simulink model "final_quadruped_230622gimbleRF"  (R2021a)
settings: Solver=ode15s  StartTime=0.0  StopTime=10  FixedStep=1e-3  RelTol=1e-5  EnableMultiTasking=on
values from neighbouring files (symbols this model uses):
  foot_x = 8    [bipedparameters.m]    (also in fcn.m; finalrobotParameters.m; finalrobotParameters_110522.m; finalrobotParameters_140522.m)
  foot_y = 6    [bipedparameters.m]    (also in fcn.m; finalrobotParameters.m; finalrobotParameters_110522.m; finalrobotParameters_140522.m)
  foot_z = 1    [bipedparameters.m]    (also in fcn.m; finalrobotParameters.m; finalrobotParameters_110522.m; finalrobotParameters_140522.m)
  height_plane = 0.025    [bipedparameters.m]    (also in finalrobotParameters.m; finalrobotParameters_110522.m; finalrobotParameters_140522.m; finalrobotParameters_240522.m)
  kd_ankle = 1000    [bipedparameters.m]    (also in finalrobotParameters_240522.m)
  kd_hip = 1000    [bipedparameters.m]    (also in finalrobotParameters_240522.m)
  kd_knee = 1000    [bipedparameters.m]    (also in finalrobotParameters_240522.m)
  ki_ankle = 1000    [bipedparameters.m]    (also in finalrobotParameters_240522.m)
  ki_hip = 1000    [bipedparameters.m]    (also in finalrobotParameters_240522.m)
  ki_knee = 2000    [bipedparameters.m]    (also in finalrobotParameters_240522.m)
  kp_ankle = 1000    [bipedparameters.m]    (also in finalrobotParameters_240522.m)
  kp_hip = 1000    [bipedparameters.m]    (also in finalrobotParameters_240522.m)
  kp_knee = 2000    [bipedparameters.m]    (also in finalrobotParameters_240522.m)
  lower_leg_length = 10    [bipedparameters.m]    (also in fcn.m; finalrobotParameters.m; finalrobotParameters_110522.m; finalrobotParameters_140522.m)
  m_ll = density*leg_radius*leg_radius*lower_leg_length*3.141592653589*0.01*0.01*0.01    (= 0.0176714586764)    [bipedparameters.m]    (also in fcn.m; finalrobotParameters_140522.m; finalrobotParameters_240522.m; hdotlb.m)
  m_ul = density*leg_radius*leg_radius*upper_leg_length*3.141592653589*0.01*0.01*0.01    (= 0.0176714586764)    [bipedparameters.m]    (also in fcn.m; finalrobotParameters_140522.m; finalrobotParameters_240522.m; hdotlb.m)
  plane_x = 25    [bipedparameters.m]    (also in finalrobotParameters.m; finalrobotParameters_110522.m; finalrobotParameters_140522.m; finalrobotParameters_240522.m)
  plane_y = 3    [bipedparameters.m]    (also in finalrobotParameters.m; finalrobotParameters_110522.m; finalrobotParameters_140522.m; finalrobotParameters_240522.m)
  torso_offset_x = -0.5    [bipedparameters.m]    (also in finalrobotParameters.m = 10; finalrobotParameters_110522.m = 10; finalrobotParameters_140522.m = 10; finalrobotParameters_240522.m = 10)
  torso_offset_z = -2    [bipedparameters.m]    (also in finalrobotParameters.m; finalrobotParameters_110522.m; finalrobotParameters_140522.m; finalrobotParameters_240522.m)
  torso_x = 5    [bipedparameters.m]    (also in fcn.m = 25; finalrobotParameters.m = 25; finalrobotParameters_110522.m = 25; finalrobotParameters_140522.m = 25)
  torso_y = 10    [bipedparameters.m]    (also in fcn.m = 16; finalrobotParameters.m = 16; finalrobotParameters_110522.m = 16; finalrobotParameters_140522.m = 16)
  torso_z = 8    [bipedparameters.m]    (also in fcn.m = 10; finalrobotParameters.m = 10; finalrobotParameters_110522.m = 10; finalrobotParameters_140522.m = 10)
  upper_leg_length = 10    [bipedparameters.m]    (also in fcn.m; finalrobotParameters.m; finalrobotParameters_110522.m; finalrobotParameters_140522.m)
undefined symbols (not defined in the file or in its folder): sigbuilder_block, X, Y, Z
libraries: nesl_utility x201, sm_lib x71, Contact_Forces_Lib x16, pid_lib x14, fl_lib x3
(part 7 of 8)

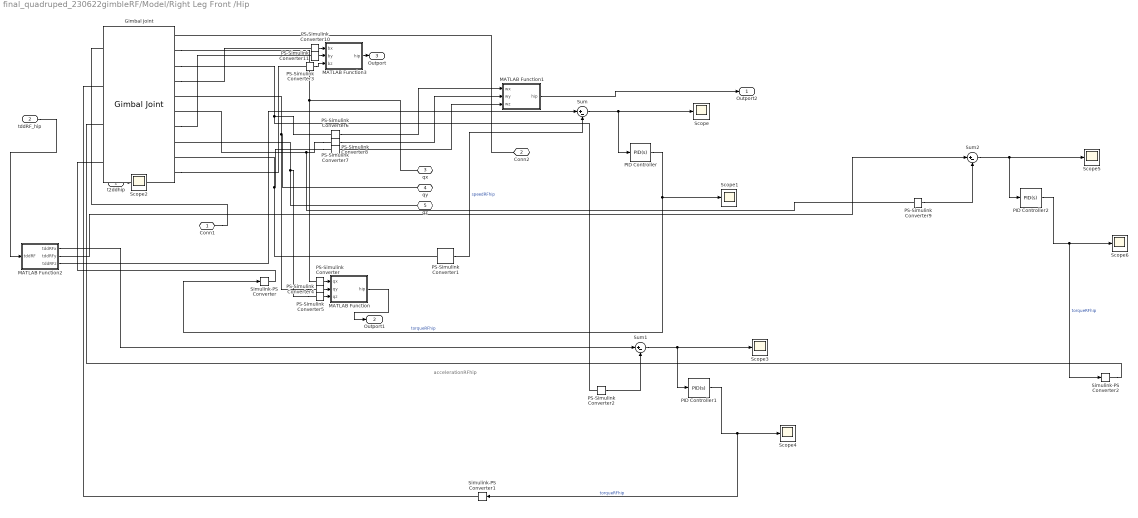
== system final_quadruped_230622gimbleRF/Model/Right Leg Front /Hip ==
  note: accelerationRFhip
  t2ddhip : Inport
  tddRF_hip : Inport  Port=2
  Gimbal Joint : sm_lib/Joints/Gimbal Joint  JointMode=Normal  SenseConstraintForce=off  SenseConstraintForceX=off  SenseConstraintForceY=off  SenseConstraintForceZ=off  SenseConstraintTorque=off  SenseConstraintTorqueX=off  SenseConstraintTorqueY=off  SenseConstraintTorqueZ=off  SenseTotalForce=off  SenseTotalForceX=off  SenseTotalForceY=off  SenseTotalForceZ=off  SenseTotalTorque=off  SenseTotalTorqueX=off  SenseTotalTorqueY=off  SenseTotalTorqueZ=off  CompositeWrenchDir=FollowerOnBase  CompositeWrenchFrame=BaseFrame  RxEquilibriumPosition=0  RxEquilibriumPositionUnits=deg  RxSpringStiffness=0  RxSpringStiffnessUnits=N*m/deg  RxDampingCoefficient=0  RxDampingCoefficientUnits=N*m/(deg/s)  RxTorqueActuationMode=InputTorque  RxMotionActuationMode=ComputedMotion  RxSensePosition=on  RxSenseVelocity=on  RxSenseAcceleration=on  RxSenseTorqueForce=off  RxSenseLowerLimitTorqueForce=off  RxSenseUpperLimitTorqueForce=off  RxLowerLimitSpecify=off  RxLowerLimitBound=-90  RxLowerLimitBoundUnits=deg  RxLowerLimitStiffness=1e4  RxLowerLimitStiffnessUnits=N*m/deg  RxLowerLimitDamping=10  RxLowerLimitDampingUnits=N*m/(deg/s)  RxLowerLimitTransitionRegionWidth=0.1  RxLowerLimitTransitionRegionWidthUnits=deg  RxUpperLimitSpecify=off  RxUpperLimitBound=90  RxUpperLimitBoundUnits=deg  RxUpperLimitStiffness=1e4  RxUpperLimitStiffnessUnits=N*m/deg  RxUpperLimitDamping=10  RxUpperLimitDampingUnits=N*m/(deg/s)  RxUpperLimitTransitionRegionWidth=0.1  RxUpperLimitTransitionRegionWidthUnits=deg  RxPositionTargetSpecify=off  RxPositionTargetPriority=High  RxPositionTargetValue=0  RxPositionTargetValueUnits=deg  RxVelocityTargetSpecify=off  RxVelocityTargetPriority=High  RxVelocityTargetValue=0  RxVelocityTargetValueUnits=deg/s  RyEquilibriumPosition=0  RyEquilibriumPositionUnits=deg  RySpringStiffness=0  RySpringStiffnessUnits=N*m/deg  RyDampingCoefficient=0  RyDampingCoefficientUnits=N*m/(deg/s)  RyTorqueActuationMode=InputTorque  RyMotionActuationMode=ComputedMotion  RySensePosition=on  RySenseVelocity=on  RySenseAcceleration=on  RySenseTorqueForce=off  RySenseLowerLimitTorqueForce=off  RySenseUpperLimitTorqueForce=off  RyLowerLimitSpecify=off  RyLowerLimitBound=-90  RyLowerLimitBoundUnits=deg  RyLowerLimitStiffness=1e4  RyLowerLimitStiffnessUnits=N*m/deg  RyLowerLimitDamping=10  RyLowerLimitDampingUnits=N*m/(deg/s)  RyLowerLimitTransitionRegionWidth=0.1  RyLowerLimitTransitionRegionWidthUnits=deg  RyUpperLimitSpecify=off  RyUpperLimitBound=90  RyUpperLimitBoundUnits=deg  RyUpperLimitStiffness=1e4  RyUpperLimitStiffnessUnits=N*m/deg  RyUpperLimitDamping=10  RyUpperLimitDampingUnits=N*m/(deg/s)  RyUpperLimitTransitionRegionWidth=0.1  RyUpperLimitTransitionRegionWidthUnits=deg  RyPositionTargetSpecify=off  RyPositionTargetPriority=High  RyPositionTargetValue=0  RyPositionTargetValueUnits=deg  RyVelocityTargetSpecify=off  RyVelocityTargetPriority=High  RyVelocityTargetValue=0  RyVelocityTargetValueUnits=deg/s  RzEquilibriumPosition=0  RzEquilibriumPositionUnits=deg  RzSpringStiffness=0  RzSpringStiffnessUnits=N*m/deg  RzDampingCoefficient=0  RzDampingCoefficientUnits=N*m/(deg/s)  RzTorqueActuationMode=InputTorque  RzMotionActuationMode=ComputedMotion  RzSensePosition=on  RzSenseVelocity=on  RzSenseAcceleration=on  RzSenseTorqueForce=off  RzSenseLowerLimitTorqueForce=off  RzSenseUpperLimitTorqueForce=off  RzLowerLimitSpecify=off  RzLowerLimitBound=-90  RzLowerLimitBoundUnits=deg  RzLowerLimitStiffness=1e4  RzLowerLimitStiffnessUnits=N*m/deg  RzLowerLimitDamping=10  RzLowerLimitDampingUnits=N*m/(deg/s)  RzLowerLimitTransitionRegionWidth=0.1  RzLowerLimitTransitionRegionWidthUnits=deg  RzUpperLimitSpecify=off  RzUpperLimitBound=90  RzUpperLimitBoundUnits=deg  RzUpperLimitStiffness=1e4  RzUpperLimitStiffnessUnits=N*m/deg  RzUpperLimitDamping=10  RzUpperLimitDampingUnits=N*m/(deg/s)  RzUpperLimitTransitionRegionWidth=0.1  RzUpperLimitTransitionRegionWidthUnits=deg  RzPositionTargetSpecify=on  RzPositionTargetPriority=Low  RzPositionTargetValue=-10  RzPositionTargetValueUnits=deg  RzVelocityTargetSpecify=on  RzVelocityTargetPriority=Low  RzVelocityTargetValue=1  RzVelocityTargetValueUnits=deg/s
  MATLAB Function : MATLAB Function  TreatAsAtomicUnit=on
  MATLAB Function1 : MATLAB Function  TreatAsAtomicUnit=on
  MATLAB Function2 : MATLAB Function  TreatAsAtomicUnit=on
  MATLAB Function3 : MATLAB Function  TreatAsAtomicUnit=on
  PID Controller : pid_lib/PID Controller  Controller=PID  Form=Parallel  TimeDomain=Continuous-time  UseExternalTs=off  SampleTime=-1  IntegratorMethod=Forward Euler  FilterMethod=Forward Euler  ControllerParametersSource=internal  P=kp_hip  I=ki_hip  D=kd_hip  UseFilter=on  N=100  TunerSelectOption=Transfer Function Based (PID Tuner App)  InitialConditionSource=internal  InitialConditionForIntegrator=0  InitialConditionForFilter=0  DifferentiatorICPrevScaledInput=0  ExternalReset=none  TrackingMode=off  Kt=1  LimitOutput=off  SatLimitsSource=internal  UpperSaturationLimit=inf  LowerSaturationLimit=-inf  LinearizeAsGain=on  AntiWindupMode=none  Kb=1  POutMin=[]  POutMax=[]  IOutMin=[]  IOutMax=[]  DOutMin=[]  DOutMax=[]  NOutMin=[]  NOutMax=[]  SumOutMin=[]  SumOutMax=[]  SaturationOutMin=[]  SaturationOutMax=[]  PParamMin=[]  PParamMax=[]  IParamMin=[]  IParamMax=[]  DParamMin=[]  DParamMax=[]  NParamMin=[]  NParamMax=[]  KbParamMin=[]  KbParamMax=[]  KtParamMin=[]  KtParamMax=[]  KbOutMin=[]  KbOutMax=[]  KtOutMin=[]  KtOutMax=[]  IntegratorOutMin=[]  IntegratorOutMax=[]  FilterOutMin=[]  FilterOutMax=[]  SumI1OutMin=[]  SumI1OutMax=[]  SumI2OutMin=[]  SumI2OutMax=[]  SumI3OutMin=[]  SumI3OutMax=[]  SumI4OutMin=[]  SumI4OutMax=[]  SumDOutMin=[]  SumDOutMax=[]  DifferentiatorOutMin=[]  DifferentiatorOutMax=[]  FilterDiffOutCoefMin=[]  FilterDiffOutCoefMax=[]  ReciprocalOutMin=[]  ReciprocalOutMax=[]  SumDenOutMin=[]  SumDenOutMax=[]  SumNumOutMin=[]  SumNumOutMax=[]  DivideOutMin=[]  DivideOutMax=[]  UdiffTsProdOutMin=[]  UdiffTsProdOutMax=[]  NTsProdOutMin=[]  NTsProdOutMax=[]  UintegralTsProdOutMin=[]  UintegralTsProdOutMax=[]  UngainTsProdOutMin=[]  UngainTsProdOutMax=[]  IntegratorContinuousStateAttributes=''  IntegratorStateMustResolveToSignalObject=off  IntegratorRTWStateStorageClass=Auto  FilterContinuousStateAttributes=''  FilterStateMustResolveToSignalObject=off  FilterRTWStateStorageClass=Auto  ParallelPVariant=InternalParameters  IdealPVariant=Disabled  IVariant=InternalParameters  DVariant=InternalParameters  IntegratorVariant=Continuous  SatVariant=Disabled  AWVariant=Passthrough  PCopyVariant=Disabled  TRVariant=Disabled  FdbkBlocksVariant=Forward  IdealPFdbkVariant=Disabled  SatFdbkVariant=Disabled  DerivativeFilterVariant=ContFilter  NVariant=InternalParameters  NCopyVariant=Disabled  FilterICVariant=InternalICsFilter  IntegratorICVariant=InternalICs  ExternalResetVariant=Disabled  TRSumVariant=Passthrough  SumFdbkVariant=Disabled  SumVariant=Sum_PID  TsampFilterVariant=InternalTs  TsampNgainVariant=Passthrough  TsampIntegralVariant=Passthrough  ExternalSaturationOutDataTypeStr=Inherit: Same as second input
  PID Controller1 : pid_lib/PID Controller  Controller=PID  Form=Parallel  TimeDomain=Continuous-time  UseExternalTs=off  SampleTime=-1  IntegratorMethod=Forward Euler  FilterMethod=Forward Euler  ControllerParametersSource=internal  P=kp_hip  I=ki_hip  D=kd_hip  UseFilter=on  N=100  TunerSelectOption=Transfer Function Based (PID Tuner App)  InitialConditionSource=internal  InitialConditionForIntegrator=0  InitialConditionForFilter=0  DifferentiatorICPrevScaledInput=0  ExternalReset=none  TrackingMode=off  Kt=1  LimitOutput=off  SatLimitsSource=internal  UpperSaturationLimit=inf  LowerSaturationLimit=-inf  LinearizeAsGain=on  AntiWindupMode=none  Kb=1  POutMin=[]  POutMax=[]  IOutMin=[]  IOutMax=[]  DOutMin=[]  DOutMax=[]  NOutMin=[]  NOutMax=[]  SumOutMin=[]  SumOutMax=[]  SaturationOutMin=[]  SaturationOutMax=[]  PParamMin=[]  PParamMax=[]  IParamMin=[]  IParamMax=[]  DParamMin=[]  DParamMax=[]  NParamMin=[]  NParamMax=[]  KbParamMin=[]  KbParamMax=[]  KtParamMin=[]  KtParamMax=[]  KbOutMin=[]  KbOutMax=[]  KtOutMin=[]  KtOutMax=[]  IntegratorOutMin=[]  IntegratorOutMax=[]  FilterOutMin=[]  FilterOutMax=[]  SumI1OutMin=[]  SumI1OutMax=[]  SumI2OutMin=[]  SumI2OutMax=[]  SumI3OutMin=[]  SumI3OutMax=[]  SumI4OutMin=[]  SumI4OutMax=[]  SumDOutMin=[]  SumDOutMax=[]  DifferentiatorOutMin=[]  DifferentiatorOutMax=[]  FilterDiffOutCoefMin=[]  FilterDiffOutCoefMax=[]  ReciprocalOutMin=[]  ReciprocalOutMax=[]  SumDenOutMin=[]  SumDenOutMax=[]  SumNumOutMin=[]  SumNumOutMax=[]  DivideOutMin=[]  DivideOutMax=[]  UdiffTsProdOutMin=[]  UdiffTsProdOutMax=[]  NTsProdOutMin=[]  NTsProdOutMax=[]  UintegralTsProdOutMin=[]  UintegralTsProdOutMax=[]  UngainTsProdOutMin=[]  UngainTsProdOutMax=[]  IntegratorContinuousStateAttributes=''  IntegratorStateMustResolveToSignalObject=off  IntegratorRTWStateStorageClass=Auto  FilterContinuousStateAttributes=''  FilterStateMustResolveToSignalObject=off  FilterRTWStateStorageClass=Auto  ParallelPVariant=InternalParameters  IdealPVariant=Disabled  IVariant=InternalParameters  DVariant=InternalParameters  IntegratorVariant=Continuous  SatVariant=Disabled  AWVariant=Passthrough  PCopyVariant=Disabled  TRVariant=Disabled  FdbkBlocksVariant=Forward  IdealPFdbkVariant=Disabled  SatFdbkVariant=Disabled  DerivativeFilterVariant=ContFilter  NVariant=InternalParameters  NCopyVariant=Disabled  FilterICVariant=InternalICsFilter  IntegratorICVariant=InternalICs  ExternalResetVariant=Disabled  TRSumVariant=Passthrough  SumFdbkVariant=Disabled  SumVariant=Sum_PID  TsampFilterVariant=InternalTs  TsampNgainVariant=Passthrough  TsampIntegralVariant=Passthrough  ExternalSaturationOutDataTypeStr=Inherit: Same as second input
  PID Controller2 : pid_lib/PID Controller  Controller=PID  Form=Parallel  TimeDomain=Continuous-time  UseExternalTs=off  SampleTime=-1  IntegratorMethod=Forward Euler  FilterMethod=Forward Euler  ControllerParametersSource=internal  P=kp_hip  I=ki_hip  D=kd_hip  UseFilter=on  N=100  TunerSelectOption=Transfer Function Based (PID Tuner App)  InitialConditionSource=internal  InitialConditionForIntegrator=0  InitialConditionForFilter=0  DifferentiatorICPrevScaledInput=0  ExternalReset=none  TrackingMode=off  Kt=1  LimitOutput=off  SatLimitsSource=internal  UpperSaturationLimit=inf  LowerSaturationLimit=-inf  LinearizeAsGain=on  AntiWindupMode=none  Kb=1  POutMin=[]  POutMax=[]  IOutMin=[]  IOutMax=[]  DOutMin=[]  DOutMax=[]  NOutMin=[]  NOutMax=[]  SumOutMin=[]  SumOutMax=[]  SaturationOutMin=[]  SaturationOutMax=[]  PParamMin=[]  PParamMax=[]  IParamMin=[]  IParamMax=[]  DParamMin=[]  DParamMax=[]  NParamMin=[]  NParamMax=[]  KbParamMin=[]  KbParamMax=[]  KtParamMin=[]  KtParamMax=[]  KbOutMin=[]  KbOutMax=[]  KtOutMin=[]  KtOutMax=[]  IntegratorOutMin=[]  IntegratorOutMax=[]  FilterOutMin=[]  FilterOutMax=[]  SumI1OutMin=[]  SumI1OutMax=[]  SumI2OutMin=[]  SumI2OutMax=[]  SumI3OutMin=[]  SumI3OutMax=[]  SumI4OutMin=[]  SumI4OutMax=[]  SumDOutMin=[]  SumDOutMax=[]  DifferentiatorOutMin=[]  DifferentiatorOutMax=[]  FilterDiffOutCoefMin=[]  FilterDiffOutCoefMax=[]  ReciprocalOutMin=[]  ReciprocalOutMax=[]  SumDenOutMin=[]  SumDenOutMax=[]  SumNumOutMin=[]  SumNumOutMax=[]  DivideOutMin=[]  DivideOutMax=[]  UdiffTsProdOutMin=[]  UdiffTsProdOutMax=[]  NTsProdOutMin=[]  NTsProdOutMax=[]  UintegralTsProdOutMin=[]  UintegralTsProdOutMax=[]  UngainTsProdOutMin=[]  UngainTsProdOutMax=[]  IntegratorContinuousStateAttributes=''  IntegratorStateMustResolveToSignalObject=off  IntegratorRTWStateStorageClass=Auto  FilterContinuousStateAttributes=''  FilterStateMustResolveToSignalObject=off  FilterRTWStateStorageClass=Auto  ParallelPVariant=InternalParameters  IdealPVariant=Disabled  IVariant=InternalParameters  DVariant=InternalParameters  IntegratorVariant=Continuous  SatVariant=Disabled  AWVariant=Passthrough  PCopyVariant=Disabled  TRVariant=Disabled  FdbkBlocksVariant=Forward  IdealPFdbkVariant=Disabled  SatFdbkVariant=Disabled  DerivativeFilterVariant=ContFilter  NVariant=InternalParameters  NCopyVariant=Disabled  FilterICVariant=InternalICsFilter  IntegratorICVariant=InternalICs  ExternalResetVariant=Disabled  TRSumVariant=Passthrough  SumFdbkVariant=Disabled  SumVariant=Sum_PID  TsampFilterVariant=InternalTs  TsampNgainVariant=Passthrough  TsampIntegralVariant=Passthrough  ExternalSaturationOutDataTypeStr=Inherit: Same as second input
  PS-Simulink Converter{,2..11} (11 alike) : nesl_utility/PS-Simulink Converter  PhysicalDomain=network_engine_domain  SubClassName=ps_output  LeftPortType=input  RightPortType=output  PseudoPeriodic=off  Frequencies=[]  Unit=inherit  AffineConversion=off
      settings: SourceProductBaseCode=PW,SS
  PS-Simulink Converter1 : nesl_utility/PS-Simulink Converter  PhysicalDomain=network_engine_domain  SubClassName=ps_output  LeftPortType=input  RightPortType=output  PseudoPeriodic=off  Frequencies=[]  Unit=1  AffineConversion=off
      settings: SourceProductBaseCode=PW,SS
  Scope{,1..6} (7 alike) : Scope
  Simulink-PS Converter : nesl_utility/Simulink-PS Converter  PhysicalDomain=network_engine_domain  SubClassName=ps_input  LeftPortType=input  RightPortType=output  PseudoPeriodic=off  Frequencies=[]  NoiseDistribution=none  NoiseParameters=[]  Unit=1  AffineConversion=off  FilteringAndDerivatives=provide  SimscapeFilterOrder=1  InputFilterTimeConstant=0.001  UdotUserProvided=0
      settings: SourceProductBaseCode=PW,SS
  Simulink-PS Converter1 : nesl_utility/Simulink-PS Converter  PhysicalDomain=network_engine_domain  SubClassName=ps_input  LeftPortType=input  RightPortType=output  PseudoPeriodic=off  Frequencies=[]  NoiseDistribution=none  NoiseParameters=[]  Unit=1  AffineConversion=off  FilteringAndDerivatives=provide  SimscapeFilterOrder=1  InputFilterTimeConstant=0.001  UdotUserProvided=0
      settings: SourceProductBaseCode=PW,SS
  Simulink-PS Converter2 : nesl_utility/Simulink-PS Converter  PhysicalDomain=network_engine_domain  SubClassName=ps_input  LeftPortType=input  RightPortType=output  PseudoPeriodic=off  Frequencies=[]  NoiseDistribution=none  NoiseParameters=[]  Unit=1  AffineConversion=off  FilteringAndDerivatives=provide  SimscapeFilterOrder=1  InputFilterTimeConstant=0.001  UdotUserProvided=0
      settings: SourceProductBaseCode=PW,SS
  Sum : Sum  Inputs=|+-
  Sum1 : Sum  Inputs=|+-
  Sum2 : Sum  Inputs=|+-
  Conn1 : PMIOPort  Side=Left
  Conn2 : PMIOPort  Port=2  Side=Right
  qx : PMIOPort  Port=3  Side=Right
  qy : PMIOPort  Port=4  Side=Right
  qz : PMIOPort  Port=5  Side=Right
  Outport2 : Outport
  Outport1 : Outport  Port=2
  Outport : Outport  Port=3
  wires:
  PS-Simulink Converter1/1 -> Sum/2  "speedRFhip"
  Sum/1 -> PID Controller/1, Scope/1
  PID Controller/1 -> Scope1/1, Simulink-PS Converter/1  "torqueRFhip"
  MATLAB Function1/1(hip) -> Outport2/1
  t2ddhip/1 -> Scope2/1
  PS-Simulink Converter/1 -> MATLAB Function/1(qx)
  PS-Simulink Converter4/1 -> MATLAB Function/2(qy)
  PS-Simulink Converter5/1 -> MATLAB Function/3(qz)
  MATLAB Function/1(hip) -> Outport1/1
  PS-Simulink Converter6/1 -> MATLAB Function1/1(wx)
  PS-Simulink Converter7/1 -> MATLAB Function1/2(wy)
  PS-Simulink Converter8/1 -> MATLAB Function1/3(wz)
  tddRF_hip/1 -> MATLAB Function2/1(tddRF)
  PID Controller1/1 -> Simulink-PS Converter1/1, Scope4/1  "torqueRFhip"
  Sum1/1 -> PID Controller1/1, Scope3/1
  MATLAB Function2/1(tddRFx) -> Sum1/1
  PS-Simulink Converter2/1 -> Sum1/2
  MATLAB Function2/3(tddRFz) -> Sum/1
  PID Controller2/1 -> Simulink-PS Converter2/1, Scope6/1  "torqueRFhip"
  Sum2/1 -> PID Controller2/1, Scope5/1
  MATLAB Function2/2(tddRFy) -> Sum2/1
  PS-Simulink Converter9/1 -> Sum2/2
  PS-Simulink Converter10/1 -> MATLAB Function3/1(bx)
  PS-Simulink Converter3/1 -> MATLAB Function3/3(bz)
  PS-Simulink Converter11/1 -> MATLAB Function3/2(by)
  MATLAB Function3/1(hip) -> Outport/1
  connections:
  Conn2/RConn1 -- Gimbal Joint/RConn1
  Conn1/RConn1 -- Gimbal Joint/LConn1
  Gimbal Joint/RConn2 -- qx/RConn1 -- PS-Simulink Converter/LConn1
  PS-Simulink Converter4/LConn1 -- Gimbal Joint/RConn5 -- qy/RConn1
  PS-Simulink Converter5/LConn1 -- Gimbal Joint/RConn8 -- qz/RConn1
  Gimbal Joint/RConn3 -- PS-Simulink Converter2/LConn1 -- PS-Simulink Converter6/LConn1
  PS-Simulink Converter7/LConn1 -- Gimbal Joint/RConn6 -- PS-Simulink Converter9/LConn1
  PS-Simulink Converter8/LConn1 -- Gimbal Joint/RConn9 -- PS-Simulink Converter1/LConn1
  Simulink-PS Converter1/RConn1 -- Gimbal Joint/LConn2
  Simulink-PS Converter2/RConn1 -- Gimbal Joint/LConn3
  Simulink-PS Converter/RConn1 -- Gimbal Joint/LConn4
  Gimbal Joint/RConn4 -- PS-Simulink Converter10/LConn1
  Gimbal Joint/RConn7 -- PS-Simulink Converter11/LConn1
  Gimbal Joint/RConn10 -- PS-Simulink Converter3/LConn1

== system final_quadruped_230622gimbleRF/Model/Right Leg Front /Knee ==
  note: accelerationRFknee
  note: Meas for knee
  tddRF_knee : Inport
  t2ddknee : Inport  Port=2
  Bus Creator : BusCreator  Inputs=3
  Knee joint : sm_lib/Joints/Revolute Joint  JointMode=Normal  SenseConstraintForce=off  SenseConstraintForceX=off  SenseConstraintForceY=off  SenseConstraintForceZ=off  SenseConstraintTorque=off  SenseConstraintTorqueX=off  SenseConstraintTorqueY=off  SenseConstraintTorqueZ=off  SenseTotalForce=off  SenseTotalForceX=off  SenseTotalForceY=off  SenseTotalForceZ=off  SenseTotalTorque=off  SenseTotalTorqueX=off  SenseTotalTorqueY=off  SenseTotalTorqueZ=off  CompositeWrenchDir=FollowerOnBase  CompositeWrenchFrame=BaseFrame  EquilibriumPosition=0  EquilibriumPositionUnits=deg  SpringStiffness=0  SpringStiffnessUnits=N*m/deg  DampingCoefficient=0  DampingCoefficientUnits=N*m/(deg/s)  TorqueActuationMode=InputTorque  MotionActuationMode=ComputedMotion  SensePosition=on  SenseVelocity=on  SenseAcceleration=on  SenseTorqueForce=off  SenseLowerLimitTorqueForce=off  SenseUpperLimitTorqueForce=off  LowerLimitSpecify=on  LowerLimitBound=0  LowerLimitBoundUnits=deg  LowerLimitStiffness=1e4  LowerLimitStiffnessUnits=N*m/deg  LowerLimitDamping=10  LowerLimitDampingUnits=N*m/(deg/s)  LowerLimitTransitionRegionWidth=0.1  LowerLimitTransitionRegionWidthUnits=deg  UpperLimitSpecify=on  UpperLimitBound=20  UpperLimitBoundUnits=deg  UpperLimitStiffness=1e4  UpperLimitStiffnessUnits=N*m/deg  UpperLimitDamping=10  UpperLimitDampingUnits=N*m/(deg/s)  UpperLimitTransitionRegionWidth=0.1  UpperLimitTransitionRegionWidthUnits=deg  PositionTargetSpecify=on  PositionTargetPriority=Low  PositionTargetValue=20  PositionTargetValueUnits=deg  VelocityTargetSpecify=on  VelocityTargetPriority=Low  VelocityTargetValue=-2  VelocityTargetValueUnits=deg/s
  PID Controller : pid_lib/PID Controller  Controller=PID  Form=Parallel  TimeDomain=Continuous-time  UseExternalTs=off  SampleTime=-1  IntegratorMethod=Forward Euler  FilterMethod=Forward Euler  ControllerParametersSource=internal  P=kp_knee  I=ki_knee  D=kd_knee  UseFilter=on  N=100  TunerSelectOption=Transfer Function Based (PID Tuner App)  InitialConditionSource=internal  InitialConditionForIntegrator=0  InitialConditionForFilter=0  DifferentiatorICPrevScaledInput=0  ExternalReset=none  TrackingMode=off  Kt=1  LimitOutput=off  SatLimitsSource=internal  UpperSaturationLimit=inf  LowerSaturationLimit=-inf  LinearizeAsGain=on  AntiWindupMode=none  Kb=1  POutMin=[]  POutMax=[]  IOutMin=[]  IOutMax=[]  DOutMin=[]  DOutMax=[]  NOutMin=[]  NOutMax=[]  SumOutMin=[]  SumOutMax=[]  SaturationOutMin=[]  SaturationOutMax=[]  PParamMin=[]  PParamMax=[]  IParamMin=[]  IParamMax=[]  DParamMin=[]  DParamMax=[]  NParamMin=[]  NParamMax=[]  KbParamMin=[]  KbParamMax=[]  KtParamMin=[]  KtParamMax=[]  KbOutMin=[]  KbOutMax=[]  KtOutMin=[]  KtOutMax=[]  IntegratorOutMin=[]  IntegratorOutMax=[]  FilterOutMin=[]  FilterOutMax=[]  SumI1OutMin=[]  SumI1OutMax=[]  SumI2OutMin=[]  SumI2OutMax=[]  SumI3OutMin=[]  SumI3OutMax=[]  SumI4OutMin=[]  SumI4OutMax=[]  SumDOutMin=[]  SumDOutMax=[]  DifferentiatorOutMin=[]  DifferentiatorOutMax=[]  FilterDiffOutCoefMin=[]  FilterDiffOutCoefMax=[]  ReciprocalOutMin=[]  ReciprocalOutMax=[]  SumDenOutMin=[]  SumDenOutMax=[]  SumNumOutMin=[]  SumNumOutMax=[]  DivideOutMin=[]  DivideOutMax=[]  UdiffTsProdOutMin=[]  UdiffTsProdOutMax=[]  NTsProdOutMin=[]  NTsProdOutMax=[]  UintegralTsProdOutMin=[]  UintegralTsProdOutMax=[]  UngainTsProdOutMin=[]  UngainTsProdOutMax=[]  IntegratorContinuousStateAttributes=''  IntegratorStateMustResolveToSignalObject=off  IntegratorRTWStateStorageClass=Auto  FilterContinuousStateAttributes=''  FilterStateMustResolveToSignalObject=off  FilterRTWStateStorageClass=Auto  ParallelPVariant=InternalParameters  IdealPVariant=Disabled  IVariant=InternalParameters  DVariant=InternalParameters  IntegratorVariant=Continuous  SatVariant=Disabled  AWVariant=Passthrough  PCopyVariant=Disabled  TRVariant=Disabled  FdbkBlocksVariant=Forward  IdealPFdbkVariant=Disabled  SatFdbkVariant=Disabled  DerivativeFilterVariant=ContFilter  NVariant=InternalParameters  NCopyVariant=Disabled  FilterICVariant=InternalICsFilter  IntegratorICVariant=InternalICs  ExternalResetVariant=Disabled  TRSumVariant=Passthrough  SumFdbkVariant=Disabled  SumVariant=Sum_PID  TsampFilterVariant=InternalTs  TsampNgainVariant=Passthrough  TsampIntegralVariant=Passthrough  ExternalSaturationOutDataTypeStr=Inherit: Same as second input
  PS-Simulink Converter : nesl_utility/PS-Simulink Converter  PhysicalDomain=network_engine_domain  SubClassName=ps_output  LeftPortType=input  RightPortType=output  PseudoPeriodic=off  Frequencies=[]  Unit=inherit  AffineConversion=off
      settings: SourceProductBaseCode=PW,SS
  PS-Simulink Converter1 : nesl_utility/PS-Simulink Converter  PhysicalDomain=network_engine_domain  SubClassName=ps_output  LeftPortType=input  RightPortType=output  PseudoPeriodic=off  Frequencies=[]  Unit=1  AffineConversion=off
      settings: SourceProductBaseCode=PW,SS
  PS-Simulink Converter2 : nesl_utility/PS-Simulink Converter  PhysicalDomain=network_engine_domain  SubClassName=ps_output  LeftPortType=input  RightPortType=output  PseudoPeriodic=off  Frequencies=[]  Unit=inherit  AffineConversion=off
      settings: SourceProductBaseCode=PW,SS
  PS-Simulink Converter3 : nesl_utility/PS-Simulink Converter  PhysicalDomain=network_engine_domain  SubClassName=ps_output  LeftPortType=input  RightPortType=output  PseudoPeriodic=off  Frequencies=[]  Unit=1  AffineConversion=off
      settings: SourceProductBaseCode=PW,SS
  Scope : Scope
  Scope1 : Scope
  Scope2 : Scope
  Simulink-PS Converter : nesl_utility/Simulink-PS Converter  PhysicalDomain=network_engine_domain  SubClassName=ps_input  LeftPortType=input  RightPortType=output  PseudoPeriodic=off  Frequencies=[]  NoiseDistribution=none  NoiseParameters=[]  Unit=1  AffineConversion=off  FilteringAndDerivatives=provide  SimscapeFilterOrder=1  InputFilterTimeConstant=0.001  UdotUserProvided=0
      settings: SourceProductBaseCode=PW,SS
  Sum : Sum  Inputs=|+-
  Conn1 : PMIOPort  Side=Left
  Conn2 : PMIOPort  Port=2  Side=Right
  q : PMIOPort  Port=3  Side=Left
  meas : Outport
  Outport : Outport  Port=2
  Outport2 : Outport  Port=3
  wires:
  Bus Creator/1 -> meas/1
  PS-Simulink Converter3/1 -> Bus Creator/1  "angleRFknee"
  PS-Simulink Converter1/1 -> Outport/1, Bus Creator/2  "speedRFknee"
  Sum/1 -> Scope1/1, PID Controller/1
  PID Controller/1 -> Bus Creator/3, Simulink-PS Converter/1, Scope/1  "torqueRFknee"
  PS-Simulink Converter2/1 -> Outport2/1
  PS-Simulink Converter/1 -> Sum/2
  t2ddknee/1 -> Scope2/1
  tddRF_knee/1 -> Sum/1
  connections:
  Knee joint/RConn2 -- q/RConn1 -- PS-Simulink Converter3/LConn1
  Knee joint/LConn1 -- Conn1/RConn1
  Conn2/RConn1 -- Knee joint/RConn1
  PS-Simulink Converter1/LConn1 -- Knee joint/RConn3 -- PS-Simulink Converter/LConn1
  Simulink-PS Converter/RConn1 -- Knee joint/LConn2
  PS-Simulink Converter2/LConn1 -- Knee joint/RConn4

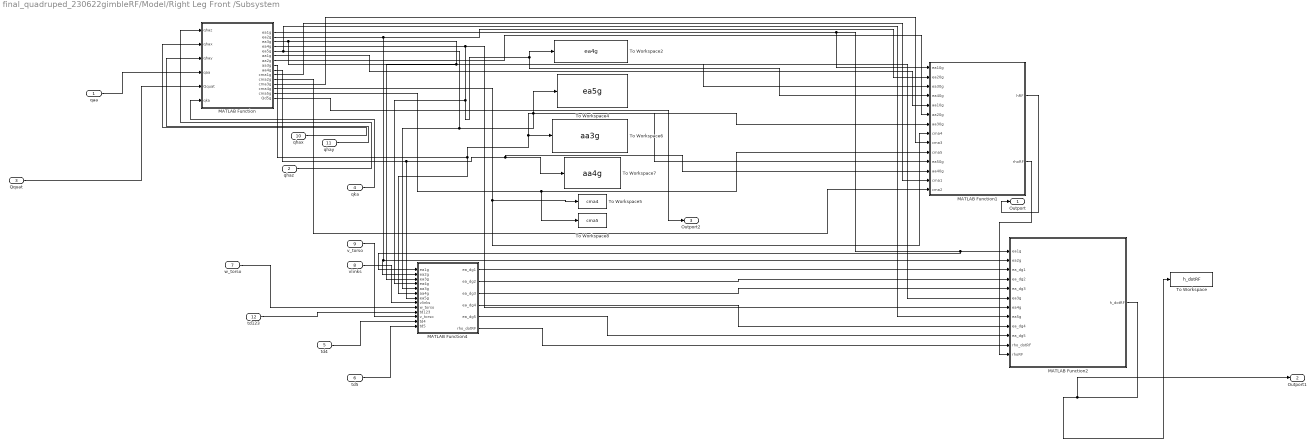
== system final_quadruped_230622gimbleRF/Model/Right Leg Front /Subsystem ==
  qaa : Inport
  qhaz : Inport  Port=2
  Qquat : Inport  Port=3
  qka : Inport  Port=4
  td4 : Inport  Port=5
  td5 : Inport  Port=6
  w_torso : Inport  Port=7
  vlinks : Inport  Port=8
  v_torso : Inport  Port=9
  qhax : Inport  Port=10
  qhay : Inport  Port=11
  td123 : Inport  Port=12
  MATLAB Function : MATLAB Function  TreatAsAtomicUnit=on
  MATLAB Function1 : MATLAB Function  TreatAsAtomicUnit=on
  MATLAB Function2 : MATLAB Function  TreatAsAtomicUnit=on
  MATLAB Function4 : MATLAB Function  TreatAsAtomicUnit=on
  To Workspace : ToWorkspace  VariableName=h_dotRF  SaveFormat=Timeseries  SampleTime=-1
  To Workspace2 : ToWorkspace  VariableName=ea4g  SaveFormat=Timeseries  SampleTime=-1
  To Workspace4 : ToWorkspace  VariableName=ea5g  SaveFormat=Timeseries  SampleTime=-1
  To Workspace5 : ToWorkspace  VariableName=cma4  SaveFormat=Timeseries  SampleTime=-1
  To Workspace6 : ToWorkspace  VariableName=aa3g  SaveFormat=Timeseries  SampleTime=-1
  To Workspace7 : ToWorkspace  VariableName=aa4g  SaveFormat=Timeseries  SampleTime=-1
  To Workspace8 : ToWorkspace  VariableName=cma5  SaveFormat=Timeseries  SampleTime=-1
  Outport : Outport
  Outport1 : Outport  Port=2
  Outport2 : Outport  Port=3
  wires:
  MATLAB Function/12(cma3g) -> MATLAB Function1/9(cma3)
  MATLAB Function/8(aa3g) -> To Workspace6/1, MATLAB Function1/7(aa30g), MATLAB Function4/6(aa4g)
  MATLAB Function/9(aa4g) -> MATLAB Function1/12(aa40g), To Workspace7/1, MATLAB Function4/7(ea5g)
  MATLAB Function/4(ea4g) -> MATLAB Function2/7(ea4g), To Workspace2/1, MATLAB Function1/4(ea40g), MATLAB Function4/4(ea4g)
  MATLAB Function/14(cma5g) -> To Workspace8/1, MATLAB Function1/10(cma5)
  MATLAB Function/3(ea3g) -> MATLAB Function2/6(ea3g), MATLAB Function4/3(ea3g), MATLAB Function1/3(ea30g)
  MATLAB Function/13(cma4g) -> MATLAB Function1/8(cma4), To Workspace5/1
  MATLAB Function/5(ea5g) -> MATLAB Function2/8(ea5g), MATLAB Function4/5(aa3g), To Workspace4/1, MATLAB Function1/11(ea50g)
  MATLAB Function1/1(hRF) -> Outport/1
  qka/1 -> MATLAB Function/6(qka)
  qaa/1 -> MATLAB Function/4(qaa)
  Qquat/1 -> MATLAB Function/5(Qquat)
  qhaz/1 -> MATLAB Function/1(qhaz)
  td123/1 -> MATLAB Function4/10(td123)
  td4/1 -> MATLAB Function4/12(td4)
  td5/1 -> MATLAB Function4/13(td5)
  vlinks/1 -> MATLAB Function4/8(vlinks)
  v_torso/1 -> MATLAB Function4/11(v_torso)
  MATLAB Function1/2(rhoRF) -> MATLAB Function2/12(rhoRF)
  MATLAB Function2/1(h_dotRF) -> To Workspace/1, Outport1/1
  MATLAB Function/15(Qd5g) -> Outport2/1
  w_torso/1 -> MATLAB Function4/9(w_torso)
  qhax/1 -> MATLAB Function/2(qhax)
  qhay/1 -> MATLAB Function/3(qhay)
  MATLAB Function/1(ea1g) -> MATLAB Function4/1(ea1g), MATLAB Function2/1(ea1g), MATLAB Function1/1(ea10g)
  MATLAB Function/2(ea2g) -> MATLAB Function2/2(ea2g), MATLAB Function4/2(ea2g), MATLAB Function1/2(ea20g)
  MATLAB Function/6(aa1g) -> MATLAB Function1/5(aa10g)
  MATLAB Function/7(aa2g) -> MATLAB Function1/6(aa20g)
  MATLAB Function/10(cma1g) -> MATLAB Function1/13(cma1)
  MATLAB Function/11(cma2g) -> MATLAB Function1/14(cma2)
  MATLAB Function4/1(ea_dg1) -> MATLAB Function2/3(ea_dg1)
  MATLAB Function4/2(ea_dg2) -> MATLAB Function2/4(ea_dg2)
  MATLAB Function4/3(ea_dg3) -> MATLAB Function2/5(ea_dg3)
  MATLAB Function4/4(ea_dg4) -> MATLAB Function2/9(ea_dg4)
  MATLAB Function4/5(ea_dg5) -> MATLAB Function2/10(ea_dg5)
  MATLAB Function4/6(rho_dotRF) -> MATLAB Function2/11(rho_dotRF)

== matlab function final_quadruped_230622gimbleRF/Model/Right Leg Front /Subsystem/MATLAB Function ==
  data: ea1g output; ea2g output; ea3g output; ea4g output; ea5g output; aa1g output; aa2g output; qhaz input; qhax input; qhay input; qaa input; Qquat input; qka input; aa3g output; aa4g output; cma1g output; cma2g output; cma3g output; cma4g output; cma5g output; Qd5g output
function [ea1g,ea2g,ea3g,ea4g,ea5g,aa1g,aa2g,aa3g,aa4g,cma1g,cma2g,cma3g,cma4g,cma5g,Qd5g] = fcn(qhaz,qhax,qhay,qaa,Qquat,qka)
%%
lower_leg_length = 10;
upper_leg_length = 10;
foot_offset=[-1; 0; 0];

%%
Qd0g=quat2rotm([Qquat(1) Qquat(2) Qquat(3) Qquat(4)]);

%x,y,z are with respect to joint's frame
%z of joint is y of robot
Qd30z=[cos(qhaz) 0 sin(qhaz);
      0 1 0 ;
      -sin(qhaz) 0 cos(qhaz)];
Qd30y=[cos(qhay) 0 sin(qhay);
      0 1 0 ;
      -sin(qhay) 0 cos(qhay)];
Qd30x=[cos(qhax) 0 sin(qhax);
      0 1 0 ;
      -sin(qhax) 0 cos(qhax)];
  
Qd30=Qd30x*Qd30y*Qd30z*Qd0g;
Qd3g=Qd30*Qd0g;
  
Qd43=[cos(qka) 0 sin(qka);
      0 1 0 ;
      -sin(qka) 0 cos(qka)];
  
Qd54=[1 0 0;
      0 cos(qaa) -sin(qaa);
      0 sin(qaa) cos(qaa)];
  
Qd40 = Qd43* Qd30;
Qd50=Qd54*Qd40;
Qd4g=Qd40*Qd0g;
Qd5g=Qd50*Qd0g;

%axis in local frames
ed1l=[1;0;0];
ed2l=[0;1;0];
ed3l=[0;
      0;
      1];
  
ed4l=[0;
      1;
      0];
ed5l=[0;
     0;
     1];
  
%link vector in local frame
ad3l=[0;
      0;
      -upper_leg_length];
   
ad4l=[0;
      0;
      -lower_leg_length];
         
%axis in global frames
ea1g=Qd30x*ed1l;
ea2g=Qd30y*ed2l;
ea3g = Qd30z*ed3l;
ea4g = Qd4g*ed4l;
ea5g = Qd5g*ed5l;

%link vector in global frame
aa1g=0;
aa2g=0;
aa3g = Qd3g*ad3l;
aa4g = Qd4g*ad4l;

%COM distances in base frame
cma1g=0;
cma2g=0;
cma3g=aa3g/2;
cma4g=aa4g/2;
cma5g=Qd5g*foot_offset;


end

== matlab function final_quadruped_230622gimbleRF/Model/Left Leg Front/Subsystem/MATLAB Function ==
  data: eb1g output; eb2g output; eb3g output; qhb input; qab input; Qquat input; qkb input; ab1g output; ab2g output; cmb1g output; cmb2g output; cmb3g output; Qd3g output
function [eb1g,eb2g,eb3g,ab1g,ab2g,cmb1g,cmb2g,cmb3g,Qd3g] = fcn(qhb,qab,Qquat,qkb)
%%
lower_leg_length = 10;
upper_leg_length = 10;
foot_offset=[-1; 0; 0];

%%
Qd10=zeros(3,3);
% disp(Qquat);
% Qquat=reshape(Qquat,4,1);
Qd0g=quat2rotm([Qquat(1) Qquat(2) Qquat(3) Qquat(4)]);
% Qd0geul=quat2eul(Qquat);
% Qd0g=eul2rotm(Qd0geul);
Qd10=[cos(qhb) 0 sin(qhb);
      0 1 0 ;
      -sin(qhb) 0 cos(qhb)];
Qd1g=Qd10*Qd0g;
  
Qd21=[cos(qkb) 0 sin(qkb);
      0 1 0 ;
      -sin(qkb) 0 cos(qkb)];
  
Qd32=[1 0 0;
      0 cos(qab) -sin(qab);
      0 sin(qab) cos(qab)];
  
Qd20 = Qd21* Qd10;
Qd30=Qd32*Qd20;
Qd2g=Qd20*Qd0g;
Qd3g=Qd30*Qd0g;

%axis in local frames
ed1l=[0;
      1;
      0];
ed2l=[0;
      1;
      0];
ed3l=[0;
     0;
     1];
  
%link vector in local frame
ad1l=[0;
      0;
      -upper_leg_length];
   
ad2l=[0;
      0;
      -lower_leg_length];
         
%axis in global frames
eb1g = Qd1g*ed1l;
eb2g = Qd2g*ed2l;
eb3g = Qd3g*ed3l;

%link vector in global frame
ab1g = Qd1g*ad1l;
ab2g = Qd2g*ad2l;

%COM distances in base frame
cmb1g=ab1g/2;
cmb2g=ab2g/2;
cmb3g=Qd3g*foot_offset;


end

== matlab function final_quadruped_230622gimbleRF/Model/Right Leg Back/Subsystem/MATLAB Function ==
  data: ec1g output; ec2g output; ec3g output; qhc input; qac input; Qquat input; qkc input; ac1g output; ac2g output; cmc1g output; cmc2g output; cmc3g output; Qd3g output
function [ec1g,ec2g,ec3g,ac1g,ac2g,cmc1g,cmc2g,cmc3g,Qd3g] = fcn(qhc,qac,Qquat,qkc)
%%
lower_leg_length = 10;
upper_leg_length = 10;
foot_offset=[-1; 0; 0];

%%
Qd0g=quat2rotm([Qquat(1) Qquat(2) Qquat(3) Qquat(4)]);
Qd10=[cos(qhc) 0 sin(qhc);
      0 1 0 ;
      -sin(qhc) 0 cos(qhc)];
Qd1g=Qd10*Qd0g;
  
Qd21=[cos(qkc) 0 sin(qkc);
      0 1 0 ;
      -sin(qkc) 0 cos(qkc)];
  
Qd32=[1 0 0;
      0 cos(qac) -sin(qac);
      0 sin(qac) cos(qac)];
  
Qd20 = Qd21* Qd10;
Qd30=Qd32*Qd20;
Qd2g=Qd20*Qd0g;
Qd3g=Qd30*Qd0g;

%axis in local frames
ed1l=[0;
      1;
      0];
ed2l=[0;
      1;
      0];
ed3l=[0;
     0;
     1];
  
%link vector in local frame
ad1l=[0;
      0;
      -upper_leg_length];
   
ad2l=[0;
      0;
      -lower_leg_length];
         
%axis in global frames
ec1g = Qd1g*ed1l;
ec2g = Qd2g*ed2l;
ec3g = Qd3g*ed3l;

%link vector in global frame
ac1g = Qd1g*ad1l;
ac2g = Qd2g*ad2l;

%COM distances in base frame
cmc1g=ac1g/2;
cmc2g=ac2g/2;
cmc3g=Qd3g*foot_offset;


end

== matlab function final_quadruped_230622gimbleRF/Model/Left LegBack/Subsystem/MATLAB Function ==
  data: ed1g output; ed2g output; ed3g output; qhd input; qad input; Qquat input; qkd input; ad1g output; ad2g output; cmd1g output; cmd2g output; cmd3g output; Qd3g output
function [ed1g,ed2g,ed3g,ad1g,ad2g,cmd1g,cmd2g,cmd3g,Qd3g] = fcn(qhd,qad,Qquat, qkd)
%%
lower_leg_length = 10;
upper_leg_length = 10;
foot_offset=[-1; 0; 0];

%%
Qd0g=quat2rotm([Qquat(1) Qquat(2) Qquat(3) Qquat(4)]);
Qd10=[cos(qhd) 0 sin(qhd);
      0 1 0 ;
      -sin(qhd) 0 cos(qhd)];
Qd1g=Qd10*Qd0g;
  
Qd21=[cos(qkd) 0 sin(qkd);
      0 1 0 ;
      -sin(qkd) 0 cos(qkd)];
  
Qd32=[1 0 0;
      0 cos(qad) -sin(qad);
      0 sin(qad) cos(qad)];
  
Qd20 = Qd21* Qd10;
Qd30=Qd32*Qd20;
Qd2g=Qd20*Qd0g;
Qd3g=Qd30*Qd0g;

%axis in local frames
ed1l=[0;
      1;
      0];
ed2l=[0;
      1;
      0];
ed3l=[0;
     0;
     1];
  
%link vector in local frame
ad1l=[0;
      0;
      -upper_leg_length];
   
ad2l=[0;
      0;
      -lower_leg_length];
         
%axis in global frames
ed1g = Qd1g*ed1l;
ed2g = Qd2g*ed2l;
ed3g = Qd3g*ed3l;

%link vector in global frame
ad1g = Qd1g*ad1l;
ad2g = Qd2g*ad2l;

%COM distances in base frame
cmd1g=ad1g/2;
cmd2g=ad2g/2;
cmd3g=Qd3g*foot_offset;


end

== matlab function final_quadruped_230622gimbleRF/Model/MATLAB Function4 ==
  data: hLF input; hRB input; hLB input; h_dotLF input; N input; hRF input; h_dotRF input; tddRF output; v_torso input; tddLF output; tddRB output; tddLB output; h output; h_dot output; h_dotRB input; t2d input; h_dotLB input; theta_d_des output; M output; t input
function [tddRF,tddLF,tddRB,tddLB,h,h_dot,theta_d_des,M] = fcn(hLF, hRB,hLB, h_dotLF, N, hRF,h_dotRF, v_torso, h_dotRB,t2d, h_dotLB,t)
%%
lower_leg_length = 10;
upper_leg_length = 10;
density = 1000;
foot_density=2000;
leg_radius = 0.75;
foot_x = 8;
foot_y = 6;
foot_z = 1;
torso_y = 16;
torso_x = 25;
torso_z = 10;
m_ul=density*leg_radius*leg_radius*upper_leg_length*3.141592653589*0.01*0.01*0.01;
m_ll=density*leg_radius*leg_radius*lower_leg_length*3.141592653589*0.01*0.01*0.01;
m_foot=foot_density*foot_x*foot_y*foot_z*0.000001;
m_torso=density*torso_x*torso_y*torso_z*0.000001;
M=m_torso+(4*(m_ul+m_ll+m_foot));
mu_s = 0.8;
%%
h=[hRF hLF hRB hLB];
h_dot=[h_dotRF h_dotLF h_dotRB h_dotLB];

% if t<0.225
%     tddfun= @(x)norm(pinv(h)*(M*[x;0;0]-M*v_torso))^2;
%     C=[1 0 0];
%     A = C*h_dot*pinv(h)*pinv(C)*M;
%     b = mu_s*N-N+C*h_dot*pinv(h)*pinv(C)*C*v_torso*M-C*h*t2d;
%     Aeq = [];
%     beq = [];
%     lb = 0;
%     ub =1;
%     x0 = 0.001;
%     options=optimoptions('fmincon', 'Algorithm', 'sqp');
%     x= fmincon(tddfun,x0,A,b,[],[],lb,ub,[],options);
% else
%     x=0.04;
% end    
    
% if t<0.05
%     theta_d_des=-pinv(h)*M*v_torso;
% else
%theta_d_des=pinv(h)*(M*[x;0;0]-M*v_torso);
theta_d_des=pinv(h)*(-M*v_torso);


tddRF_hipx=theta_d_des(1);
tddRF_hipy=theta_d_des(2);
tddRF_hipz=theta_d_des(3);
tddRF_knee=theta_d_des(4);
tddRF_ankle=theta_d_des(5);
tddLF_hip=theta_d_des(6);
tddLF_knee=theta_d_des(7);
tddLF_ankle=theta_d_des(8);
tddRB_hip=theta_d_des(9);
tddRB_knee=theta_d_des(10);
tddRB_ankle=theta_d_des(11);
tddLB_hip=theta_d_des(12);
tddLB_knee=theta_d_des(13);
tddLB_ankle=theta_d_des(14);

tddRF=[tddRF_hipx tddRF_hipy tddRF_hipz tddRF_knee tddRF_ankle];
tddLF=[tddLF_hip tddLF_knee tddLF_ankle];
tddRB=[tddRB_hip tddRB_knee tddRB_ankle];
tddLB=[tddLB_hip tddLB_knee tddLB_ankle];
end

== matlab function final_quadruped_230622gimbleRF/Model/Right Leg Front /Subsystem/MATLAB Function1 ==
  data: ea10g input; ea20g input; ea30g input; ea40g input; aa10g input; aa20g input; aa30g input; cma4 input; cma3 input; cma5 input; ea50g input; aa40g input; hRF output; rhoRF output; cma1 input; cma2 input
function [hRF,rhoRF] = fcn(ea10g,ea20g,ea30g, ea40g,aa10g,aa20g, aa30g, cma4, cma3, cma5, ea50g, aa40g,cma1,cma2)
%%
lower_leg_length = 10;
upper_leg_length = 10;
density = 1000;
foot_density=2000;
leg_radius = 0.75;
foot_x = 8;
foot_y = 6;
foot_z = 1;
m_ul=density*leg_radius*leg_radius*upper_leg_length*3.141592653589*0.01*0.01*0.01;
m_ll=density*leg_radius*leg_radius*lower_leg_length*3.141592653589*0.01*0.01*0.01;
m_foot=foot_density*foot_x*foot_y*foot_z*0.000001;
m1=0;
m2=0;
%%
scf=zeros(3,5);
sof=zeros(3,5);
rhoRF=zeros(3,5,5);
scf(:,1)=[0;0;0];
scf(:,2)=[0;0;0];
scf(:,3)=cma3;
scf(:,4)=aa30g+cma4;
scf(:,5)=aa30g+aa40g+cma5;
sof(:,1)=[0;0;0];
sof(:,2)=[0;0;0];
sof(:,3)=[0;0;0];
sof(:,4)=aa30g;
sof(:,5)=aa30g+aa40g;
for i=1:5
    for j=1:5
        if j<i
rhoRF(:,j,i)=zeros(3,1);
        else
rhoRF(:,j,i)=scf(:,j)-sof(:,i);
        end
    end
end
h1=m1*(cross(ea10g,rhoRF(:,1,1)))+m2*(cross(ea10g,rhoRF(:,2,1)))+m_ul*(cross(ea10g,rhoRF(:,3,1)))+m_ll*(cross(ea10g,rhoRF(:,4,1)))+m_foot*(cross(ea10g,rhoRF(:,5,1)));
h2=m2*(cross(ea20g,rhoRF(:,2,2)))+m_ul*(cross(ea20g,rhoRF(:,3,2)))+m_ll*(cross(ea20g,rhoRF(:,4,2)))+m_foot*(cross(ea20g,rhoRF(:,5,2)));
h3=(m_ul*cross(ea30g,rhoRF(:,3,3)))+(m_ll*cross(ea30g,rhoRF(:,4,3)))+(m_foot*cross(ea30g,rhoRF(:,5,3)));
h4=(m_ll*cross(ea40g,rhoRF(:,4,4)))+(m_foot*cross(ea40g,rhoRF(:,5,4)));
h5=m_foot*(cross(ea50g,rhoRF(:,5,5)));

hRF =[h1 h2 h3 h4 h5];



end

== matlab function final_quadruped_230622gimbleRF/Model/Left Leg Front/Subsystem/MATLAB Function1 ==
  data: eb10g input; eb20g input; ab10g input; cmb2 input; cmb1 input; cmb3 input; eb30g input; hLF output; ab20g input; rhoLF output
function [hLF,rhoLF] = fcn(eb10g, eb20g, ab10g, cmb2, cmb1, cmb3, eb30g, ab20g)
%%
lower_leg_length = 10;
upper_leg_length = 10;
density = 1000;
foot_density=2000;
leg_radius = 0.75;
foot_x = 8;
foot_y = 6;
foot_z = 1;
m_ul=density*leg_radius*leg_radius*upper_leg_length*3.141592653589*0.01*0.01*0.01;
m_ll=density*leg_radius*leg_radius*lower_leg_length*3.141592653589*0.01*0.01*0.01;
m_foot=foot_density*foot_x*foot_y*foot_z*0.000001;
%%
scf=zeros(3,3);
sof=zeros(3,3);
rhoLF=zeros(3,3,3);
scf(:,1)=cmb1;
scf(:,2)=ab10g+cmb2;
scf(:,3)=ab10g+ab20g+cmb3;
sof(:,1)=[0;0;0];
sof(:,2)=ab10g;
sof(:,3)=ab10g+ab20g;
for i=1:3
    for j=1:3
        if j<i
rhoLF(:,j,i)=zeros(3,1);
        else
rhoLF(:,j,i)=scf(:,j)-sof(:,i);
        end
    end
end
h1=(m_ul*cross(eb10g,rhoLF(:,1,1)))+(m_ll*cross(eb10g,rhoLF(:,2,1)))+(m_foot*cross(eb10g,rhoLF(:,3,1)));
h2=(m_ll*cross(eb20g,rhoLF(:,2,2)))+(m_foot*cross(eb20g,rhoLF(:,3,2)));
h3=m_foot*(cross(eb30g,rhoLF(:,3,3)));

hLF =[h1 h2 h3];



end

== matlab function final_quadruped_230622gimbleRF/Model/Right Leg Back/Subsystem/MATLAB Function1 ==
  data: ec10g input; ec20g input; ac10g input; cmc2 input; cmc1 input; cmc3 input; ec30g input; ac20g input; hRB output; rhoRB output
function [hRB,rhoRB] = fcn(ec10g, ec20g, ac10g, cmc2, cmc1, cmc3, ec30g, ac20g)
%%
lower_leg_length = 10;
upper_leg_length = 10;
density = 1000;
foot_density=2000;
leg_radius = 0.75;
foot_x = 8;
foot_y = 6;
foot_z = 1;
m_ul=density*leg_radius*leg_radius*upper_leg_length*3.141592653589*0.01*0.01*0.01;
m_ll=density*leg_radius*leg_radius*lower_leg_length*3.141592653589*0.01*0.01*0.01;
m_foot=foot_density*foot_x*foot_y*foot_z*0.000001;
%%
scf=zeros(3,3);
sof=zeros(3,3);
rhoRB=zeros(3,3,3);
scf(:,1)=cmc1;
scf(:,2)=ac10g+cmc2;
scf(:,3)=ac10g+ac20g+cmc3;
sof(:,1)=[0;0;0];
sof(:,2)=ac10g;
sof(:,3)=ac10g+ac20g;
for i=1:3
    for j=1:3
        if j<i
rhoRB(:,j,i)=zeros(3,1);
        else
rhoRB(:,j,i)=scf(:,j)-sof(:,i);
        end
    end
end
h1=(m_ul*cross(ec10g,rhoRB(:,1,1)))+(m_ll*cross(ec10g,rhoRB(:,2,1)))+(m_foot*cross(ec10g,rhoRB(:,3,1)));
h2=(m_ll*cross(ec20g,rhoRB(:,2,2)))+(m_foot*cross(ec20g,rhoRB(:,3,2)));
h3=m_foot*(cross(ec30g,rhoRB(:,3,3)));

hRB =[h1 h2 h3];



end

== matlab function final_quadruped_230622gimbleRF/Model/Left LegBack/Subsystem/MATLAB Function1 ==
  data: ed10g input; ed20g input; ad10g input; cmd2 input; cmd1 input; cmd3 input; ed30g input; ad20g input; hLB output; rhoLB output
function [hLB,rhoLB] = fcn(ed10g, ed20g, ad10g, cmd2, cmd1, cmd3, ed30g, ad20g)
%%
lower_leg_length = 10;
upper_leg_length = 10;
density = 1000;
foot_density=2000;
leg_radius = 0.75;
foot_x = 8;
foot_y = 6;
foot_z = 1;
m_ul=density*leg_radius*leg_radius*upper_leg_length*3.141592653589*0.01*0.01*0.01;
m_ll=density*leg_radius*leg_radius*lower_leg_length*3.141592653589*0.01*0.01*0.01;
m_foot=foot_density*foot_x*foot_y*foot_z*0.000001;
%%
scf=zeros(3,3);
sof=zeros(3,3);
rhoLB=zeros(3,3,3);
scf(:,1)=cmd1;
scf(:,2)=ad10g+cmd2;
scf(:,3)=ad10g+ad20g+cmd3;
sof(:,1)=[0;0;0];
sof(:,2)=ad10g;
sof(:,3)=ad10g+ad20g;
for i=1:3
    for j=1:3
        if j<i
rhoLB(:,j,i)=zeros(3,1);
        else
rhoLB(:,j,i)=scf(:,j)-sof(:,i);
        end
    end
end
h1=(m_ul*cross(ed10g,rhoLB(:,1,1)))+(m_ll*cross(ed10g,rhoLB(:,2,1)))+(m_foot*cross(ed10g,rhoLB(:,3,1)));
h2=(m_ll*cross(ed20g,rhoLB(:,2,2)))+(m_foot*cross(ed20g,rhoLB(:,3,2)));
h3=m_foot*(cross(ed30g,rhoLB(:,3,3)));

hLB =[h1 h2 h3];



end

== matlab function final_quadruped_230622gimbleRF/MATLAB Function ==
  data: vx input; v_torso output; vy input; vz input
function v_torso = fcn(vx, vy, vz)
v_torso=[vx; vy; vz];
end

== matlab function final_quadruped_230622gimbleRF/Model/Right Leg Front /MATLAB Function2 ==
  data: tddRF input; tddRF_hip output; tddRF_knee output; tddRF_ankle output
function [tddRF_hip, tddRF_knee, tddRF_ankle] = fcn(tddRF)
tddRF_hip=[tddRF(1);tddRF(2);tddRF(3)];
tddRF_knee=tddRF(4);
tddRF_ankle=tddRF(5);
end

== matlab function final_quadruped_230622gimbleRF/Model/Left Leg Front/MATLAB Function2 ==
  data: tddLF input; tddLF_hip output; tddLF_knee output; tddLF_ankle output
function [tddLF_hip, tddLF_knee, tddLF_ankle] = fcn(tddLF)
tddLF_hip=tddLF(1);
tddLF_knee=tddLF(2);
tddLF_ankle=tddLF(3);
end

== matlab function final_quadruped_230622gimbleRF/Model/Right Leg Back/MATLAB Function2 ==
  data: tddRB input; tddRB_hip output; tddRB_knee output; tddRB_ankle output
function [tddRB_hip, tddRB_knee, tddRB_ankle] = fcn(tddRB)
tddRB_hip=tddRB(1);
tddRB_knee=tddRB(2);
tddRB_ankle=tddRB(3);
end

== matlab function final_quadruped_230622gimbleRF/Subsystem/MATLAB Function1 ==
  data: px input; py input; pz input; p output; vx input; vy input; v output; vz input; ax input; ay input; az input; a output
function [p,v,a] = fcn(px,py,pz,vx,vy,vz,ax,ay,az)
p=[px;py;pz];
v=[vx;vy;vz];
a=[ax;ay;az];
end

== matlab function final_quadruped_230622gimbleRF/Model/Left LegBack/MATLAB Function2 ==
  data: tddLB input; tddLB_hip output; tddLB_knee output; tddLB_ankle output
function [tddLB_hip, tddLB_knee, tddLB_ankle] = fcn(tddLB)
tddLB_hip=tddLB(1);
tddLB_knee=tddLB(2);
tddLB_ankle=tddLB(3);
end

== matlab function final_quadruped_230622gimbleRF/Subsystem/MATLAB Function4 ==
  data: px input; py input; pz input; p output; vx input; vy input; v output; vz input; ax input; ay input; az input; a output
function [p,v,a] = fcn(px,py,pz,vx,vy,vz,ax,ay,az)
p=[px;py;pz];
v=[vx;vy;vz];
a=[ax;ay;az];
end

== matlab function final_quadruped_230622gimbleRF/Subsystem/MATLAB Function5 ==
  data: px input; py input; pz input; p output; vx input; vy input; v output; vz input; ax input; ay input; az input; a output
function [p,v,a] = fcn(px,py,pz,vx,vy,vz,ax,ay,az)
p=[px;py;pz];
v=[vx;vy;vz];
a=[ax;ay;az];
end

== matlab function final_quadruped_230622gimbleRF/Subsystem/MATLAB Function6 ==
  data: px input; py input; pz input; p output; vx input; vy input; v output; vz input; ax input; ay input; az input; a output
function [p,v,a] = fcn(px,py,pz,vx,vy,vz,ax,ay,az)
p=[px;py;pz];
v=[vx;vy;vz];
a=[ax;ay;az];
end

== matlab function final_quadruped_230622gimbleRF/Subsystem/MATLAB Function7 ==
  data: px input; py input; pz input; p output; vx input; vy input; v output; vz input; ax input; ay input; az input; a output
function [p,v,a] = fcn(px,py,pz,vx,vy,vz,ax,ay,az)
p=[px;py;pz];
v=[vx;vy;vz];
a=[ax;ay;az];
end

== matlab function final_quadruped_230622gimbleRF/Subsystem/MATLAB Function8 ==
  data: px input; py input; pz input; p output; vx input; vy input; v output; vz input; ax input; ay input; az input; a output
function [p,v,a] = fcn(px,py,pz,vx,vy,vz,ax,ay,az)
p=[px;py;pz];
v=[vx;vy;vz];
a=[ax;ay;az];
end

== matlab function final_quadruped_230622gimbleRF/Subsystem/MATLAB Function9 ==
  data: px input; py input; pz input; p output; vx input; vy input; v output; vz input; ax input; ay input; az input; a output
function [p,v,a] = fcn(px,py,pz,vx,vy,vz,ax,ay,az)
p=[px;py;pz];
v=[vx;vy;vz];
a=[ax;ay;az];
end

== matlab function final_quadruped_230622gimbleRF/Subsystem/MATLAB Function10 ==
  data: px input; py input; pz input; p output; vx input; vy input; v output; vz input; ax input; ay input; az input; a output
function [p,v,a] = fcn(px,py,pz,vx,vy,vz,ax,ay,az)
p=[px;py;pz];
v=[vx;vy;vz];
a=[ax;ay;az];
end

== matlab function final_quadruped_230622gimbleRF/Subsystem/MATLAB Function11 ==
  data: px input; py input; pz input; p output; vx input; vy input; v output; vz input; ax input; ay input; az input; a output
function [p,v,a] = fcn(px,py,pz,vx,vy,vz,ax,ay,az)
p=[px;py;pz];
v=[vx;vy;vz];
a=[ax;ay;az];
end

== matlab function final_quadruped_230622gimbleRF/Subsystem/MATLAB Function12 ==
  data: px input; py input; pz input; p output; vx input; vy input; v output; vz input; ax input; ay input; az input; a output
function [p,v,a] = fcn(px,py,pz,vx,vy,vz,ax,ay,az)
p=[px;py;pz];
v=[vx;vy;vz];
a=[ax;ay;az];
end

== matlab function final_quadruped_230622gimbleRF/Subsystem/MATLAB Function14 ==
  data: px input; py input; pz input; p output; vx input; vy input; v output; vz input; ax input; ay input; az input; a output
function [p,v,a] = fcn(px,py,pz,vx,vy,vz,ax,ay,az)
p=[px;py;pz];
v=[vx;vy;vz];
a=[ax;ay;az];
end
